simulink model "flyback_converter"  (Simulink 7.5)
settings: Solver=ode23tb  StartTime=0.0  StopTime=10.0  MaxStep=1e-4  RelTol=1e-3
libraries: powerlib x10, simulink x2
settings Model: Creator=mustafasyyd  LastModifiedBy=mustafasyyd

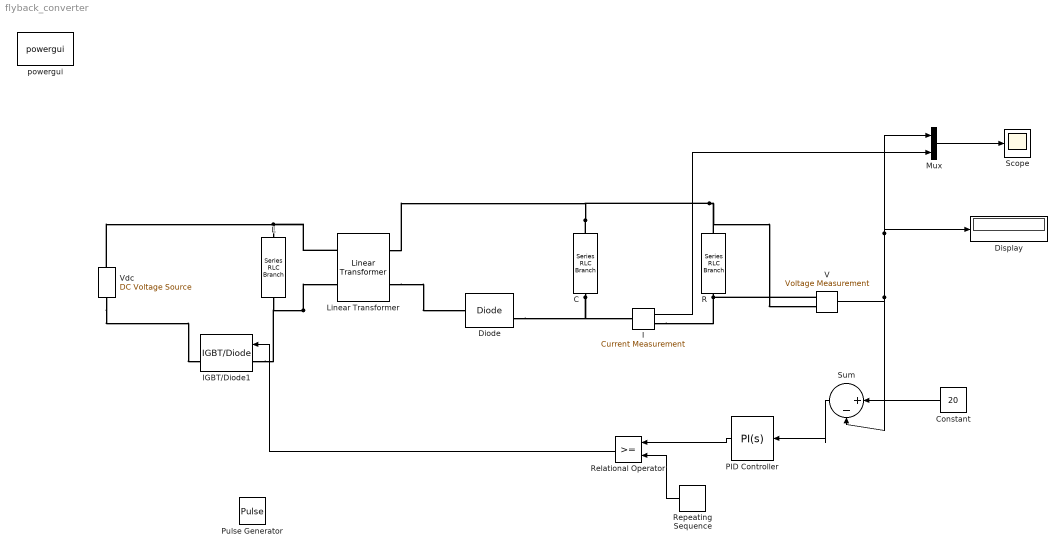
== system flyback_converter ==
  C : powerlib/Elements/Series RLC Branch  DialogController=POWERSYS.PowerSysDialog  PhysicalDomain=powersysdomain  SubClassName=unknown  LeftPortType=p1  RightPortType=p1  LConnTagsString=__new0  RConnTagsString=__new0  BranchType=C  Resistance=1  Inductance=1e-3  SetiL0=off  InitialCurrent=0  Capacitance=100e-6  Setx0=off  InitialVoltage=0  Measurements=None
  Constant : Constant  Value=20  OutDataType=fixdt(1, 16)  OutScaling=2^0
  Diode : powerlib/Power Electronics/Diode  DialogController=POWERSYS.PowerSysDialog  SystemSampleTime=-1  Ron=0.001  Lon=0  Vf=0.8  IC=0  UseSnubber=off  Rs=500  Cs=250e-9  Measurements=on
  Display : Display
  I : powerlib/Measurements/Current Measurement  DialogController=POWERSYS.PowerSysDialog  SystemSampleTime=-1  PhasorSimulation=off  OutputType=Complex  PSBequivalent=0
  IGBT/Diode1 : powerlib/Power Electronics/IGBT//Diode  DialogController=POWERSYS.PowerSysDialog  SystemSampleTime=-1  Ron=1e-3  Rs=1e5  Cs=inf  Measurements=on
  L : powerlib/Elements/Series RLC Branch  DialogController=POWERSYS.PowerSysDialog  PhysicalDomain=powersysdomain  SubClassName=unknown  LeftPortType=p1  RightPortType=p1  LConnTagsString=__new0  RConnTagsString=__new0  BranchType=L  Resistance=1  Inductance=1e-3  SetiL0=off  InitialCurrent=0  Capacitance=1e-6  Setx0=off  InitialVoltage=0  Measurements=None
  Linear Transformer : powerlib/Elements/Linear Transformer  DialogController=POWERSYS.PowerSysDialog  PhysicalDomain=powersysdomain  SubClassName=unknown  LeftPortType=p1  RightPortType=p1  LConnTagsString=a|b  RConnTagsString=A|B  UNITS=pu  NominalPower=[ 3e3 5e3 ]  winding1=[ 200 0 0 ]  winding2=[ 100 0 0]  ThreeWindings=off  RmLm=[ 500 500 ]  Measurements=None  DataType=off
  Mux : Mux  Inputs=2
  PID Controller : simulink/Continuous/PID Controller  DialogController=pidpack.PIDConfig.pidDDGCreate  DialogControllerArgs=DataTag0  SystemSampleTime=-1  Controller=PI  TimeDomain=Continuous-time  SampleTime=1  IntegratorMethod=Forward Euler  FilterMethod=Forward Euler  Form=Parallel  P=1  I=100  D=0  N=100  InitialConditionSource=internal  InitialConditionForIntegrator=0  InitialConditionForFilter=0  ExternalReset=none  LimitOutput=off  UpperSaturationLimit=inf  LowerSaturationLimit=-inf  LinearizeAsGain=off  AntiWindupMode=none  Kb=1  TrackingMode=off  Kt=1  PParamMin=[]  PParamMax=[]  IParamMin=[]  IParamMax=[]  DParamMin=[]  DParamMax=[]  NParamMin=[]  NParamMax=[]  KbParamMin=[]  KbParamMax=[]  KtParamMin=[]  KtParamMax=[]  POutMin=[]  POutMax=[]  IOutMin=[]  IOutMax=[]  DOutMin=[]  DOutMax=[]  NOutMin=[]  NOutMax=[]  KbOutMin=[]  KbOutMax=[]  KtOutMin=[]  KtOutMax=[]  IntegratorOutMin=[]  IntegratorOutMax=[]  FilterOutMin=[]  FilterOutMax=[]  SumOutMin=[]  SumOutMax=[]  SumI1OutMin=[]  SumI1OutMax=[]  SumI2OutMin=[]  SumI2OutMax=[]  SumI3OutMin=[]  SumI3OutMax=[]  SumDOutMin=[]  SumDOutMax=[]  SaturationOutMin=[]  SaturationOutMax=[]  IntegratorContinuousStateAttributes=''  IntegratorStateMustResolveToSignalObject=off  IntegratorRTWStateStorageClass=Auto  FilterContinuousStateAttributes=''  FilterStateMustResolveToSignalObject=off  FilterRTWStateStorageClass=Auto
  Pulse Generator : DiscretePulseGenerator  PulseType=Time based  Amplitude=1  Period=1/5000  PulseWidth=20  PhaseDelay=0  SampleTime=1
  R : powerlib/Elements/Series RLC Branch  DialogController=POWERSYS.PowerSysDialog  PhysicalDomain=powersysdomain  SubClassName=unknown  LeftPortType=p1  RightPortType=p1  LConnTagsString=__new0  RConnTagsString=__new0  BranchType=R  Resistance=10  Inductance=1e-3  SetiL0=off  InitialCurrent=0  Capacitance=1e-6  Setx0=off  InitialVoltage=0  Measurements=None
  Relational Operator : RelationalOperator  LogicOutDataTypeMode=boolean  LogicDataType=fixdt(0, 8)  OutDataTypeStr=boolean
  Repeating Sequence : simulink/Sources/Repeating Sequence  SystemSampleTime=-1  rep_seq_t=[0 2]  rep_seq_y=[0 2]
  Scope : Scope
      settings: YMin=0  YMax=100
  Sum : Sum  Inputs=|+-  OutDataType=fixdt(1, 16)  OutScaling=2^0
  V : powerlib/Measurements/Voltage Measurement  DialogController=POWERSYS.PowerSysDialog  SystemSampleTime=-1  PhasorSimulation=off  OutputType=Complex  PSBequivalent=0
  Vdc : powerlib/Electrical Sources/DC Voltage Source  DialogController=POWERSYS.PowerSysDialog  SystemSampleTime=-1  Amplitude=100  Measurements=None
  powergui : powerlib/powergui  Priority=1  SystemSampleTime=-1  SimulationMode=Continuous  SampleTime=50e-6  frequency=60  SPID=off  DisableSnubberDevices=off  DisableRonSwitches=off  DisableVfSwitches=off  SwTol=0  Interpol=off  frequencyindice=0  echomessages=off  HookPort=off  DisplayEquations=off  FunctionMessages=off  EnableUseOfTLC=off  x0status=blocks  RestoreLinks=warning  ResistiveCurrentMeasurement=off  Ylog=off  Xlog=on  ShowGrid=off  save=off  variable=ZData  ZoomFFT=off  StartTime=0.0  cycles=1  DisplayStyle=1  FreqAxis=off  MaxFrequency=1000  frequencyindicesteady=1  display=off  methode=off
  wires:
  V/1 -> Display/1, Mux/1, Sum/2
  Mux/1 -> Scope/1
  Sum/1 -> PID Controller/1
  Constant/1 -> Sum/1
  I/1 -> Mux/2
  PID Controller/1 -> Relational Operator/1
  Repeating Sequence/1 -> Relational Operator/2
  Relational Operator/1 -> IGBT/Diode1/1
  connections:
  L/RConn1 -- IGBT/Diode1/LConn1 -- Linear Transformer/LConn2
  R/RConn1 -- C/RConn1 -- Linear Transformer/RConn1 -- V/LConn2
  L/LConn1 -- Vdc/RConn1 -- Linear Transformer/LConn1
  Vdc/LConn1 -- IGBT/Diode1/RConn1
  Linear Transformer/RConn2 -- Diode/LConn1
  C/LConn1 -- I/LConn1 -- Diode/RConn1
  V/LConn1 -- R/LConn1 -- I/RConn1
